simulink model "Model_26_01_1"  (R2024b)
settings: Solver=FixedStepAuto  StartTime=0.0  StopTime=100  FixedStep=1e-3  RelTol=1e-3
values from neighbouring files (symbols this model uses):
  MPend_opt = parameters(MPend_opt)    [Code_26_01.m]
settings Model: Creator=traba  LastModifiedBy=chiar

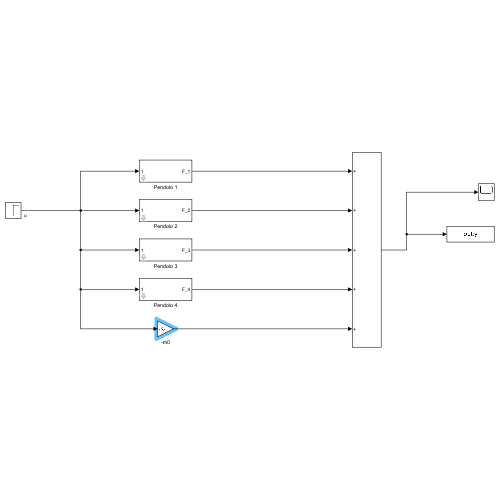
[thumbnail: Simulink's stored preview of the top-level diagram]
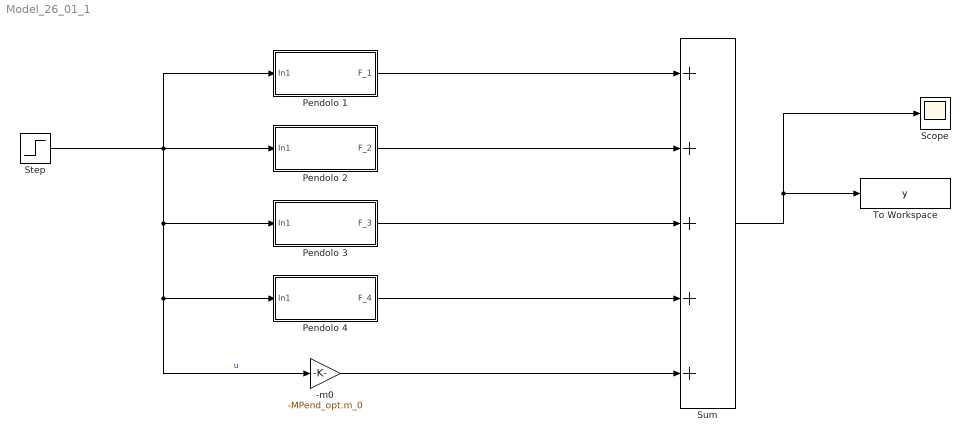
== system Model_26_01_1 ==
  -m0 : Gain  Gain=-MPend_opt.m_0
  Pendolo 1 : Subsystem  mask{n=1}
      mask prompts: n "slosh mode 1"
  Pendolo 2 : Subsystem  mask{n=2}
      mask prompts: n "slosh mode 1"
  Pendolo 3 : Subsystem  mask{n=3}
      mask prompts: n "slosh mode 1"
  Pendolo 4 : Subsystem  mask{n=3}
      mask prompts: n "slosh mode 1"
  Scope : Scope
  Step : Step  Time=0  SampleTime=0
  Sum : Sum  Inputs=+++++
  To Workspace : ToWorkspace  VariableName=y  SampleTime=-1
      settings: Save2DSignal=2-D array (concatenate along first dimension)
  wires:
  Step/1 -> Pendolo 2/1(In1), Pendolo 4/1(In1), -m0/1, Pendolo 3/1(In1), Pendolo 1/1(In1)  "u"
  Sum/1 -> Scope/1, To Workspace/1
  Pendolo 1/1(F_1) -> Sum/1
  Pendolo 2/1(F_2) -> Sum/2
  Pendolo 3/1(F_3) -> Sum/3
  Pendolo 4/1(F_4) -> Sum/4
  -m0/1 -> Sum/5

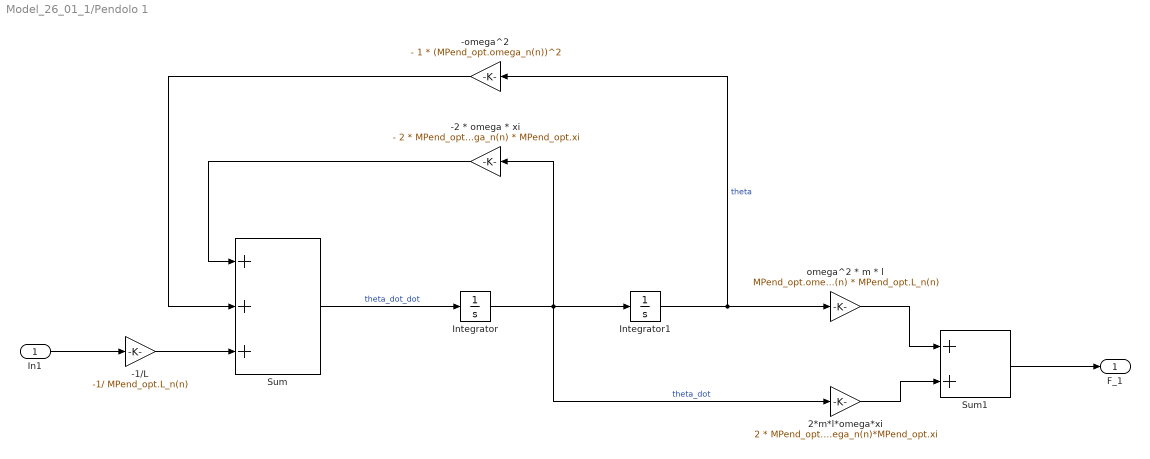
== system Model_26_01_1/Pendolo 1 ==
  In1 : Inport
  -1/L : Gain  Gain=-1/ MPend_opt.L_n(n)
  -2 * omega * xi : Gain  Gain=- 2 * MPend_opt.omega_n(n) * MPend_opt.xi
  -omega^2 : Gain  Gain=- 1 * (MPend_opt.omega_n(n))^2
  2*m*l*omega*xi : Gain  Gain=2 * MPend_opt.m_n(n)*MPend_opt.L_n(n)*MPend_opt.omega_n(n)*MPend_opt.xi
  Integrator : Integrator
  Integrator1 : Integrator
  Sum : Sum  Inputs=+++
  Sum1 : Sum
  omega^2 * m * l : Gain  Gain="MPend_opt.omega_n(n)^2 *  MPend_opt.m_n(n) * MPend_opt.L_n(n)"
  F_1 : Outport
  wires:
  Sum/1 -> Integrator/1  "theta_dot_dot"
  Integrator/1 -> 2*m*l*omega*xi/1, -2 * omega * xi/1, Integrator1/1  "theta_dot"
  -omega^2/1 -> Sum/2
  -2 * omega * xi/1 -> Sum/1
  Integrator1/1 -> omega^2 * m * l/1, -omega^2/1  "theta"
  Sum1/1 -> F_1/1
  In1/1 -> -1/L/1
  -1/L/1 -> Sum/3
  omega^2 * m * l/1 -> Sum1/1
  2*m*l*omega*xi/1 -> Sum1/2

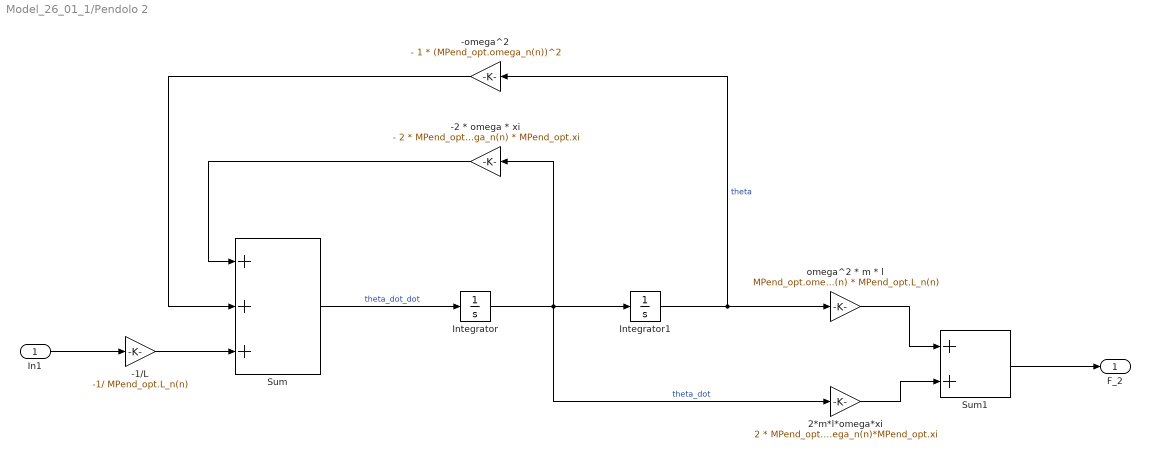
== system Model_26_01_1/Pendolo 2 ==
  In1 : Inport
  -1/L : Gain  Gain=-1/ MPend_opt.L_n(n)
  -2 * omega * xi : Gain  Gain=- 2 * MPend_opt.omega_n(n) * MPend_opt.xi
  -omega^2 : Gain  Gain=- 1 * (MPend_opt.omega_n(n))^2
  2*m*l*omega*xi : Gain  Gain=2 * MPend_opt.m_n(n)*MPend_opt.L_n(n)*MPend_opt.omega_n(n)*MPend_opt.xi
  Integrator : Integrator
  Integrator1 : Integrator
  Sum : Sum  Inputs=+++
  Sum1 : Sum
  omega^2 * m * l : Gain  Gain="MPend_opt.omega_n(n)^2 *  MPend_opt.m_n(n) * MPend_opt.L_n(n)"
  F_2 : Outport
  wires:
  Sum/1 -> Integrator/1  "theta_dot_dot"
  Integrator/1 -> 2*m*l*omega*xi/1, -2 * omega * xi/1, Integrator1/1  "theta_dot"
  -omega^2/1 -> Sum/2
  -2 * omega * xi/1 -> Sum/1
  Integrator1/1 -> omega^2 * m * l/1, -omega^2/1  "theta"
  Sum1/1 -> F_2/1
  In1/1 -> -1/L/1
  -1/L/1 -> Sum/3
  omega^2 * m * l/1 -> Sum1/1
  2*m*l*omega*xi/1 -> Sum1/2

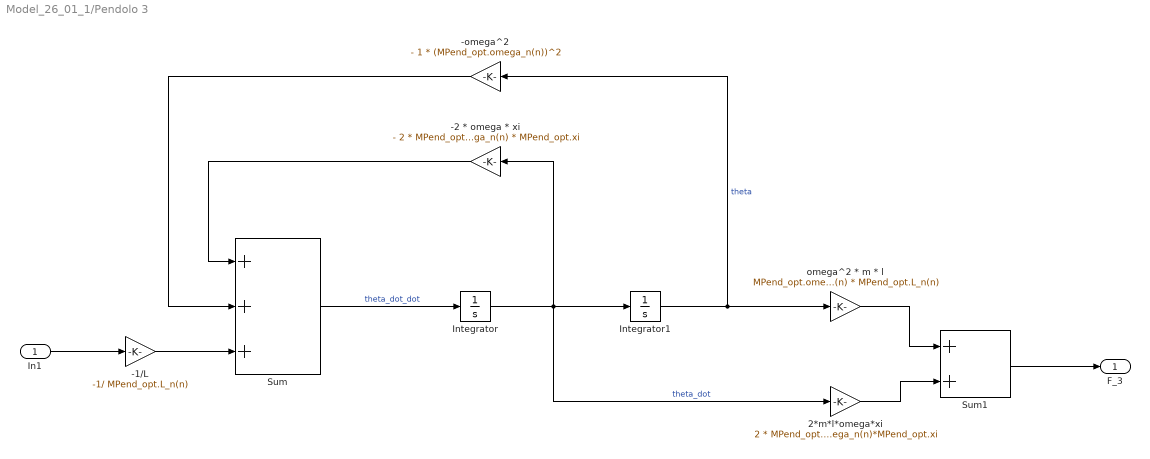
== system Model_26_01_1/Pendolo 3 ==
  In1 : Inport
  -1/L : Gain  Gain=-1/ MPend_opt.L_n(n)
  -2 * omega * xi : Gain  Gain=- 2 * MPend_opt.omega_n(n) * MPend_opt.xi
  -omega^2 : Gain  Gain=- 1 * (MPend_opt.omega_n(n))^2
  2*m*l*omega*xi : Gain  Gain=2 * MPend_opt.m_n(n)*MPend_opt.L_n(n)*MPend_opt.omega_n(n)*MPend_opt.xi
  Integrator : Integrator
  Integrator1 : Integrator
  Sum : Sum  Inputs=+++
  Sum1 : Sum
  omega^2 * m * l : Gain  Gain="MPend_opt.omega_n(n)^2 *  MPend_opt.m_n(n) * MPend_opt.L_n(n)"
  F_3 : Outport
  wires:
  Sum/1 -> Integrator/1  "theta_dot_dot"
  Integrator/1 -> 2*m*l*omega*xi/1, -2 * omega * xi/1, Integrator1/1  "theta_dot"
  -omega^2/1 -> Sum/2
  -2 * omega * xi/1 -> Sum/1
  Integrator1/1 -> omega^2 * m * l/1, -omega^2/1  "theta"
  Sum1/1 -> F_3/1
  In1/1 -> -1/L/1
  -1/L/1 -> Sum/3
  omega^2 * m * l/1 -> Sum1/1
  2*m*l*omega*xi/1 -> Sum1/2

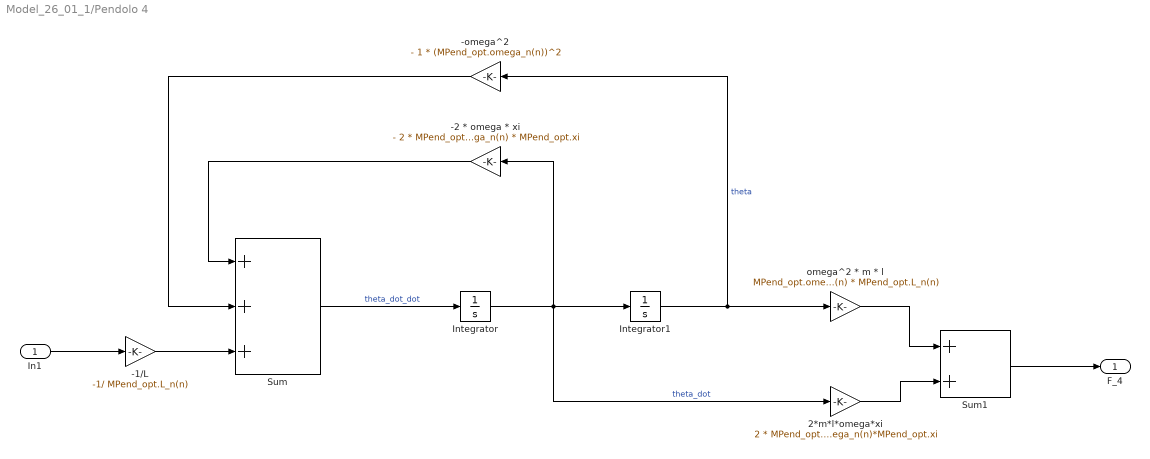
== system Model_26_01_1/Pendolo 4 ==
  In1 : Inport
  -1/L : Gain  Gain=-1/ MPend_opt.L_n(n)
  -2 * omega * xi : Gain  Gain=- 2 * MPend_opt.omega_n(n) * MPend_opt.xi
  -omega^2 : Gain  Gain=- 1 * (MPend_opt.omega_n(n))^2
  2*m*l*omega*xi : Gain  Gain=2 * MPend_opt.m_n(n)*MPend_opt.L_n(n)*MPend_opt.omega_n(n)*MPend_opt.xi
  Integrator : Integrator
  Integrator1 : Integrator
  Sum : Sum  Inputs=+++
  Sum1 : Sum
  omega^2 * m * l : Gain  Gain="MPend_opt.omega_n(n)^2 *  MPend_opt.m_n(n) * MPend_opt.L_n(n)"
  F_4 : Outport
  wires:
  Sum/1 -> Integrator/1  "theta_dot_dot"
  Integrator/1 -> 2*m*l*omega*xi/1, -2 * omega * xi/1, Integrator1/1  "theta_dot"
  -omega^2/1 -> Sum/2
  -2 * omega * xi/1 -> Sum/1
  Integrator1/1 -> omega^2 * m * l/1, -omega^2/1  "theta"
  Sum1/1 -> F_4/1
  In1/1 -> -1/L/1
  -1/L/1 -> Sum/3
  omega^2 * m * l/1 -> Sum1/1
  2*m*l*omega*xi/1 -> Sum1/2
